simulink model "deg_120_trig"  (Simulink 5.0)
settings: Solver=ode45  StartTime=0.0  StopTime=1.0  RelTol=1e-3
settings Model: LastModifiedBy=dsplab  ConsistencyChecking=warning  BlockReductionOpt=off  BooleanDataType=off

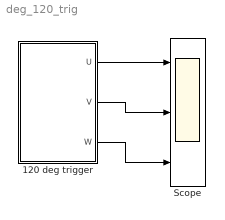
== system deg_120_trig ==
  120 deg trigger : Subsystem  mask{T=1/10, V=160}
      mask prompts: T "Time period"; V "Excitation Voltage"
  Scope : Scope  NumInputPorts=3
      settings: YMin=-5~-5~-5  YMax=5~5~5
  wires:
  120 deg trigger/1(U) -> Scope/1
  120 deg trigger/2(V) -> Scope/2
  120 deg trigger/3(W) -> Scope/3

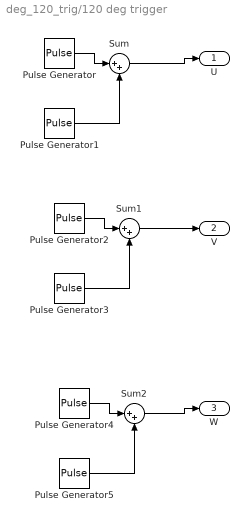
== system deg_120_trig/120 deg trigger ==
  Pulse Generator : DiscretePulseGenerator  PulseType=Time based  Amplitude=V  Period=T  PulseWidth=200/3  PhaseDelay=T/3
  Pulse Generator1 : DiscretePulseGenerator  PulseType=Time based  Amplitude=-2*V  Period=2*T  PulseWidth=100/3  PhaseDelay=-2*T/3
  Pulse Generator2 : DiscretePulseGenerator  PulseType=Time based  Amplitude=V  Period=T  PulseWidth=200/3
  Pulse Generator3 : DiscretePulseGenerator  PulseType=Time based  Amplitude=-2*V  Period=2*T  PulseWidth=100/3
  Pulse Generator4 : DiscretePulseGenerator  PulseType=Time based  Amplitude=V  Period=T  PulseWidth=200/3  PhaseDelay=-T/3
  Pulse Generator5 : DiscretePulseGenerator  PulseType=Time based  Amplitude=-2*V  Period=2*T  PulseWidth=100/3  PhaseDelay=2*T/3
  Sum : Sum  Inputs=|++  SaturateOnIntegerOverflow=on  InputSameDT=on
  Sum1 : Sum  Inputs=|++  SaturateOnIntegerOverflow=on  InputSameDT=on
  Sum2 : Sum  Inputs=|++  SaturateOnIntegerOverflow=on  InputSameDT=on
  U : Outport
  V : Outport  Port=2
  W : Outport  Port=3
  wires:
  Pulse Generator/1 -> Sum/1
  Pulse Generator1/1 -> Sum/2
  Pulse Generator2/1 -> Sum1/1
  Pulse Generator3/1 -> Sum1/2
  Pulse Generator4/1 -> Sum2/1
  Pulse Generator5/1 -> Sum2/2
  Sum/1 -> U/1
  Sum1/1 -> V/1
  Sum2/1 -> W/1
